simulink subsystem "integrator"  (R2026a)
settings: Solver=VariableStepAuto
model mask{Mass=0, Inertia=0, Pos=0, Velocity=0, Orient=0, AngVelocity=0}
  mask prompts: Mass "Mass [kg]"; Inertia "Inertia matrix (3x3)"; Pos "Initial Position (NED)"; Velocity "Initial velocity (BODY)"; Orient "Initial Orientation (NED)"; AngVelocity "Angular velocity (BODY)"
undefined symbols (not defined in the file): integrator_step
settings Model: Creator=User  LastModifiedBy=User

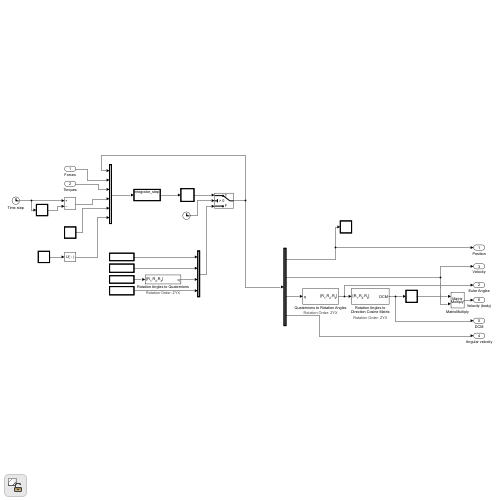
[thumbnail: Simulink's stored preview of the top-level diagram]
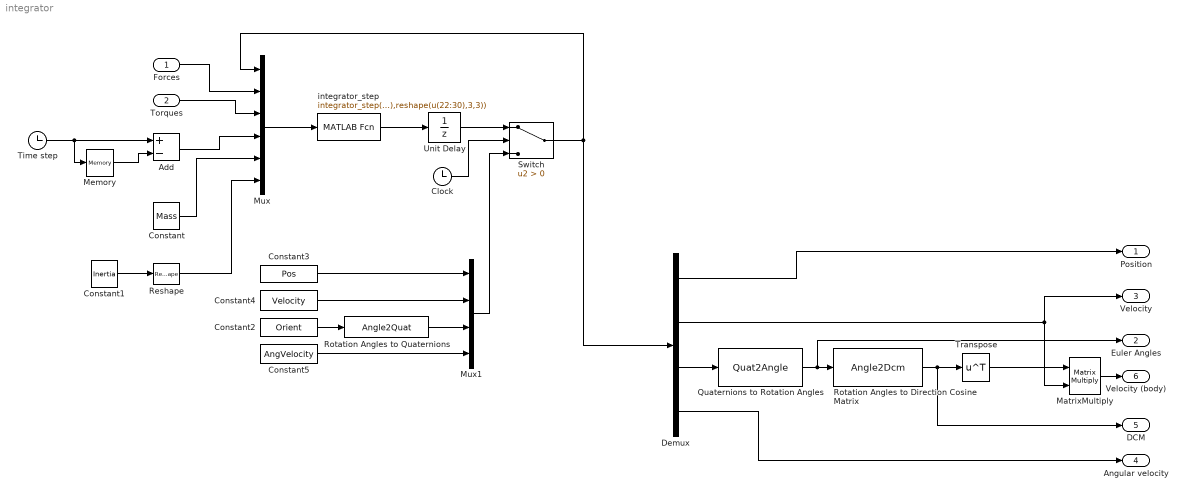
== system integrator ==
  Forces : Inport
  Torques : Inport  Port=2
  Add : Sum  Inputs=+-
  Clock : Clock
  Constant : Constant  Value=Mass
  Constant1 : Constant  Value=Inertia
  Constant2 : Constant  Value=Orient
  Constant3 : Constant  Value=Pos
  Constant4 : Constant  Value=Velocity
  Constant5 : Constant  Value=AngVelocity
  Demux : Demux  Outputs=[3 3 4 3]
  MatrixMultiply : Product  Multiplication=Matrix(*)
  Memory : Memory
  Mux : Mux  Inputs=[13 3 3 1 1 9]
  Mux1 : Mux  Inputs=[3 3 4 3]
  Quaternions to Rotation Angles : Quat2Angle
      settings: AttributesFormatString=Rotation Order: %<rotationOrder>
  Reshape : Reshape
  Rotation Angles to Direction Cosine Matrix : Angle2Dcm
      settings: AttributesFormatString=Rotation Order: %<rotationOrder>
  Rotation Angles to Quaternions : Angle2Quat
      settings: AttributesFormatString=Rotation Order: %<rotationOrder>
  Switch : Switch  Criteria=u2 > Threshold  SaturateOnIntegerOverflow=off  InputSameDT=off
  Time step : Clock
  Transpose : Math  Operator=transpose
  Unit Delay : UnitDelay  SampleTime=-1
  integrator_step : MATLABFcn  MATLABFcn=integrator_step(u(1:13),u(14:16),u(17:19),u(20),u(21),reshape(u(22:30),3,3))  OutputDimensions=[13 1]  Output1D=off
  Position : Outport
  Euler Angles : Outport  Port=2
  Velocity : Outport  Port=3
  Angular velocity : Outport  Port=4
  DCM : Outport  Port=5
  Velocity (body) : Outport  Port=6
  wires:
  integrator_step/1 -> Unit Delay/1
  Mux/1 -> integrator_step/1
  Forces/1 -> Mux/2
  Torques/1 -> Mux/3
  Time step/1 -> Memory/1, Add/1
  Memory/1 -> Add/2
  Add/1 -> Mux/4
  Constant/1 -> Mux/5
  Constant1/1 -> Reshape/1
  Constant2/1 -> Rotation Angles to Quaternions/1
  Constant3/1 -> Mux1/1
  Rotation Angles to Quaternions/1 -> Mux1/3
  Constant4/1 -> Mux1/2
  Constant5/1 -> Mux1/4
  Mux1/1 -> Switch/3
  Switch/1 -> Demux/1, Mux/1
  Clock/1 -> Switch/2
  Demux/1 -> Position/1
  Quaternions to Rotation Angles/1 -> Rotation Angles to Direction Cosine Matrix/1, Euler Angles/1
  Demux/2 -> Velocity/1, MatrixMultiply/2
  Demux/4 -> Angular velocity/1
  Transpose/1 -> MatrixMultiply/1
  Reshape/1 -> Mux/6
  Unit Delay/1 -> Switch/1
  Demux/3 -> Quaternions to Rotation Angles/1
  Rotation Angles to Direction Cosine Matrix/1 -> DCM/1, Transpose/1
  MatrixMultiply/1 -> Velocity (body)/1
